simulink model "BBB_AHRS_IMU_MARG_v2_Live"  (R2013a)
settings: Solver=FixedStepDiscrete  StartTime=0.0  StopTime=inf  FixedStep=0.01  RelTol=1e-3
libraries: BLACKlink x3, simulink_extras x3, vrlib x1
settings Model: SimulationMode=external  ExtModeTrigDuration=100  Creator=rdustinkahawita  LastModifiedBy=rdustinkahawita
settings OptimizationCC: OptimizeModelRefInitCode=on  LifeSpan=1
settings DebuggingCC: SolverPrmCheckMsg=none  StrictBusMsg=Warning
settings HardwareCC: ProdLargestAtomicInteger=Long  ProdLargestAtomicFloat=Double  ProdEndianess=LittleEndian  ProdHWDeviceType=ARM Compatible->ARM Cortex
settings RTWCC: SystemTargetFile=realtime.tlc  GenerateMakefile=off  TemplateMakefile=realtime.tmf  Description=Run on Target Hardware  RTWVerbose=off  ProcessScript=realtime_make_rtw_hook
settings STFCustomTargetCC: TargetLibSuffix=.a  GenerateSampleERTMain=on  ERTCustomFileBanners=on  SupportNonInlinedSFcns=off  SupportVariableSizeSignals=on  MATLABClassNameForMDSCustomization=Simulink.SoftwareTarget.ERTCustomization  SystemTargetFile=realtime.tlc
settings ERTTargetCC: ParMdlRefBuildCompliant=off  CompOptLevelCompliant=off  ConcurrentExecutionCompliant=off  CombineOutputUpdateFcns=off  ERTFirstTimeCompliant=off  SupportContinuousTime=on  SupportVariableSizeSignals=on  ModelStepFunctionPrototypeControlCompliant=off  CPPClassGenCompliant=off  ExtMode=on  ExtModeMexArgs='192.168.7.2' 0 17725  ERTSrcFileBannerTemplate=realtime_code_template.cgt  ERTHdrFileBannerTemplate=realtime_code_template.cgt  ERTDataSrcFileTemplate=realtime_code_template.cgt  ERTDataHdrFileTemplate=realtime_code_template.cgt  ERTCustomFileTemplate=realtime_file_process.tlc

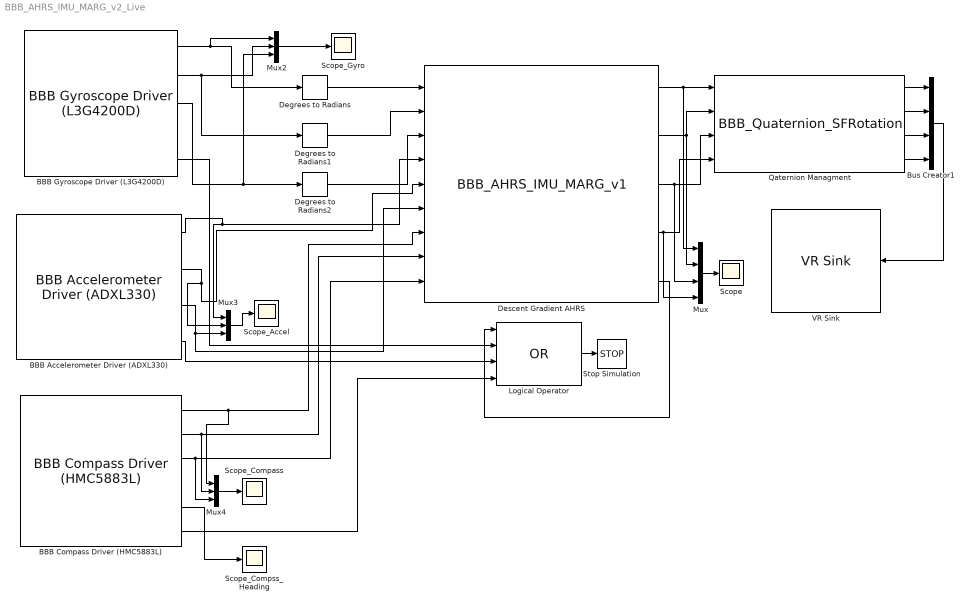
== system BBB_AHRS_IMU_MARG_v2_Live ==
  BBB Accelerometer Driver (ADXL330) : BLACKlink/BBB Accelerometer Driver (ADXL330)  BBB_AccelSensitivity=Sensitivity: 333 mV/g -> 3.3V Operating Voltage  BBB_CalibrationReq=on  BBB_DebugInfo=No Debug Info
  BBB Compass Driver (HMC5883L) : BLACKlink/BBB Compass Driver (HMC5883L)  BBB_I2CBus=BeagleBone Black I2C Channel 1  BBB_I2CAddress=Compass Address: 0x1E  BBB_Compass_DataOutAvrg=1 Sample per Measurement Output  BBB_Compass_DataOutRate=75 Hz  BBB_Compass_MeasureMode=Normal Configuration  BBB_Compass_GainValue=GN3 - Sensor Field Range: +/- 2.50 Ga; Gain: 660 LSb/Gauss  BBB_Compass_OpMode=Continuous Measurement Mode  BBB_Compass_HeadingMode=Output True North  BBB_Compass_HeadingOffset=0.0  BBB_Compass_DeclinationAng=-14.66  BBB_Compass_SelfTest=on  BBB_Compass_SelfTest_GainValue=GN0 - Sensor Field Range: +/- 0.88 Ga; Gain: 1370 LSb/Gauss  BBB_Debug_InfoLevel=No Debug Info
  "BBB Gyroscope Driver (L3G4200D) " : BLACKlink/BBB Gyroscope Driver (L3G4200D)   BBB_I2CBus=BeagleBone Black I2C Channel 1  BBB_I2CAddress=Gyro Address: 0x068  BBB_GyroRange=Range: 250 deg/sec  BBB_DebugInfo=No Debug Info
  Bus Creator1 : BusCreator
  Degrees to Radians : simulink_extras/Transformations/Degrees to Radians
  Degrees to Radians1 : simulink_extras/Transformations/Degrees to Radians
  Degrees to Radians2 : simulink_extras/Transformations/Degrees to Radians
  Descent Gradient AHRS : S-Function  InitFcn=try, set_param(gcb,'FunctionName','BBB_AHRS_IMU_MARG_v1'), end  FunctionName=BBB_AHRS_IMU_MARG_v1  SFunctionModules=BBB_AHRS_IMU_MARG_v1_wrapper  EnableBusSupport=off  mask(S-Function Builder){}
      mask help: Simulink:masks:SFunctionBuilder_MD
      mask init:
      | val = [[.9  0.75 0.75 1 1 .9 .9 1]',[1 1 0.75 0.75 .9 .9 1 .9]'];try , sys = get_param(gcb,'SfunBuilderFcnName');if isempty(sys), sys = get_param(gcb,'FunctionName'); end,catch, sys = get_param(gcb,'FunctionName'); end
      settings: CopyFcn=set_param(gcbh,'LinkStatus','none')  PreSaveFcn=try, set_param(gcb,'FunctionName','BBB_AHRS_IMU_MARG_v1'), end  OpenFcn=sfunctionwizard(gcbh)
      mask Display: plot(val(:,1),val(:,2)),disp(sys), port_label('input',1,'inGyro_w_x'), port_label('input',2,'inGyro_w_y'), port_label('input',3,'inGyro_w_z'), port_label('input',4,'inAccel_a_x'), port_label('input',5,'inAccel_a_y'), port_label('input',6,'inAccel_a_z'), port_label('input',7,'inCompass_m_x'), port_label('input',8,'inCompass_m_y'), port_label('input',9,'inCompass_m_z'), port_label('output',1,'outQuat_q_1'), port_label('output',2,'outQuat_q_2'), port_label('output',3,'outQuat_q_3'), port_label('output',4,'outQuat_q_4'), port_label('output',5,'outStopSim')
  Logical Operator : Logic  Operator=OR  Inputs=4  AllPortsSameDT=off  OutDataTypeStr=boolean
  Mux : Mux
  Mux2 : Mux  Inputs=3
  Mux3 : Mux  Inputs=3
  Mux4 : Mux  Inputs=3
  Qaternion Managment : S-Function  InitFcn=try, set_param(gcb,'FunctionName','BBB_Quaternion_SFRotation'), end  FunctionName=BBB_Quaternion_SFRotation  SFunctionModules=BBB_Quaternion_SFRotation_wrapper  EnableBusSupport=off  mask(S-Function Builder){}
      mask help: Simulink:masks:SFunctionBuilder_MD
      mask init: same as BBB_AHRS_IMU_MARG_v2_Live/Descent Gradient AHRS
      settings: CopyFcn=set_param(gcbh,'LinkStatus','none')  PreSaveFcn=try, set_param(gcb,'FunctionName','BBB_Quaternion_SFRotation'), end  OpenFcn=sfunctionwizard(gcbh)
      mask Display: plot(val(:,1),val(:,2)),disp(sys), port_label('input',1,'inQuat_q_1'), port_label('input',2,'inQuat_q_2'), port_label('input',3,'inQuat_q_3'), port_label('input',4,'inQuat_q_4'), port_label('output',1,'outSFRot_r_1'), port_label('output',2,'outSFRot_r_2'), port_label('output',3,'outSFRot_r_3'), port_label('output',4,'outSFRot_r_4')
  Scope : Scope
      settings: YMin=-0.4  YMax=1
  Scope_Accel : Scope
      settings: SaveName=ScopeData3
  Scope_Compass : Scope
      settings: YMin=-30  YMax=20  SaveName=ScopeData4
  Scope_Compss_Heading : Scope
      settings: YMin=0  YMax=375
  Scope_Gyro : Scope
      settings: YMin=-300  YMax=275  SaveName=ScopeData2
  Stop Simulation : Stop
  VR Sink : vrlib/VR Sink  InstantiateOnLoad=on  SampleTime=-1  ViewEnable=on  RemoteChange=off  RemoteView=off  FieldsWritten=BBB_Aircraft.rotation.4.1.1.double  WorldFileName=Software_Quadrotor_VRML\BBB_Plane.WRL  AutoView=off  VideoDimensions=[]  AllowVariableSize=off
  wires:
  "BBB Gyroscope Driver (L3G4200D) "/1 -> Mux2/1, Degrees to Radians/1
  "BBB Gyroscope Driver (L3G4200D) "/2 -> Mux2/2, Degrees to Radians1/1
  "BBB Gyroscope Driver (L3G4200D) "/3 -> Mux2/3, Degrees to Radians2/1
  BBB Accelerometer Driver (ADXL330)/1 -> Mux3/1, Descent Gradient AHRS/4
  BBB Accelerometer Driver (ADXL330)/2 -> Descent Gradient AHRS/5, Mux3/2
  BBB Accelerometer Driver (ADXL330)/3 -> Descent Gradient AHRS/6, Mux3/3
  Descent Gradient AHRS/5 -> Logical Operator/1
  BBB Accelerometer Driver (ADXL330)/4 -> Logical Operator/3
  Logical Operator/1 -> Stop Simulation/1
  Mux/1 -> Scope/1
  Mux2/1 -> Scope_Gyro/1
  "BBB Gyroscope Driver (L3G4200D) "/5 -> Logical Operator/2
  Degrees to Radians/1 -> Descent Gradient AHRS/1
  Degrees to Radians1/1 -> Descent Gradient AHRS/2
  Degrees to Radians2/1 -> Descent Gradient AHRS/3
  BBB Compass Driver (HMC5883L)/1 -> Mux4/1, Descent Gradient AHRS/7
  BBB Compass Driver (HMC5883L)/2 -> Mux4/2, Descent Gradient AHRS/8
  BBB Compass Driver (HMC5883L)/3 -> Mux4/3, Descent Gradient AHRS/9
  BBB Compass Driver (HMC5883L)/6 -> Logical Operator/4
  Mux3/1 -> Scope_Accel/1
  Mux4/1 -> Scope_Compass/1
  Qaternion Managment/2 -> Bus Creator1/2
  Qaternion Managment/3 -> Bus Creator1/3
  Qaternion Managment/4 -> Bus Creator1/4
  BBB Compass Driver (HMC5883L)/5 -> Scope_Compss_Heading/1
  Qaternion Managment/1 -> Bus Creator1/1
  Bus Creator1/1 -> VR Sink/1
  Descent Gradient AHRS/1 -> Qaternion Managment/1, Mux/1
  Descent Gradient AHRS/2 -> Qaternion Managment/2, Mux/2
  Descent Gradient AHRS/3 -> Mux/3, Qaternion Managment/3
  Descent Gradient AHRS/4 -> Mux/4, Qaternion Managment/4
